simulink model "DinamicaNonLineare"  (R2020b)
settings: Solver=FixedStepDiscrete  StartTime=0.0  StopTime=inf  FixedStep=0.002  RelTol=1e-3
undefined symbols (not defined in the file or in its folder): DiscIntNeverNeededParam
libraries: simulink x4, sm_lib x4, nesl_utility x4, arduinolib x1
settings Model: SILPILModeSetting=veronly  ExtModeTrigDuration=2  Creator=Tommaso  LastModifiedBy=Tommaso
settings OptimizationCC: EnhancedBackFolding=on  PassReuseOutputArgsAs=Individual arguments  ZeroExternalMemoryAtStartup=off  ZeroInternalMemoryAtStartup=off  MaxStackSize=64  OptimizeBlockOrder=speed  DifferentSizesBufferReuse=on  OptimizationCustomize=off  EfficientTunableParamExpr=on
settings DebuggingCC: ParameterTunabilityLossMsg=error
settings HardwareCC: ProdBitPerInt=16  ProdBitPerPointer=16  ProdBitPerSizeT=16  ProdBitPerPtrDiffT=16  ProdLargestAtomicFloat=None  ProdWordSize=8  ProdHWDeviceType=Atmel->AVR
settings SFSimCC: MATLABDynamicMemAlloc=off
settings RTWCC: Description=Embedded Coder  SystemTargetFile=ert.tlc  HardwareBoard=Arduino Uno  TemplateMakefile=ert_default_tmf  Toolchain=Arduino AVR
settings CodeAppCC: ForceParamTrailComments=on  IgnoreCustomStorageClasses=off  OperatorAnnotations=on  SimulinkDataObjDesc=on  SFDataObjDesc=on  InsertBlockDesc=on
settings ERTTargetCC: SupportContinuousTime=on  SupportVariableSizeSignals=on  ExtModeStaticAllocSize=250
settings ExplorerConfigSet: InternalSimMechanicsExplorerSettings="<ExplorerConfiguration><canonicalview>default</canonicalview><AnimationSetting><BasePlaybackSpeed>1.0</BasePlaybackSpeed><PlaybackSpeedFactor>1.0</PlaybackSpeedFactor></AnimationSetting><TilePanel><TileInfo><Tiles Columns=\"1\" Count=\"1\" Rows=\"1\"><Column Weight=\"1\"/><Row Weight=\"1\"/><Tile Height=\"1\" Width=\"1\" X=\"0\" Y=\"0\"/></Tiles></TileInfo><SceneInfo><SceneViewer><BGColor><R>0.60000002384185791</R><G>0.60000002384185791</G><B>0.60000002384185791</B></BGColor><Camera><DoPerspective>off</DoPerspective><Position><X>-0.0398988425731658936</X><Y>-1.00037544965744019</Y><Z>0.00866047292947813574</Z></Position><Center><X>-0.0398988425731658936</X><Y>-0.000375449657440185547</Y><Z>0.00866047292947813574</Z></Center><Up><X>0</X><Y>-0</Y><Z>1</Z></Up><ViewLimDist>1</ViewLimDist><YLim>0.125903869368592103</YLim><XLim>0.183246225714683547</XLim></Camera></SceneViewer></SceneInfo></TilePanel><MechEditorPanel><Cameras/><GfxPanelCameraMap/><VideoCreator><PlaybackSpeedRatio>1.0</PlaybackSpeedRatio><FrameRate>30</FrameRate><VideoFormat>Motion JPEG AVI</VideoFormat><FrameSize>auto</FrameSize></VideoCreator></MechEditorPanel></ExplorerConfiguration>"

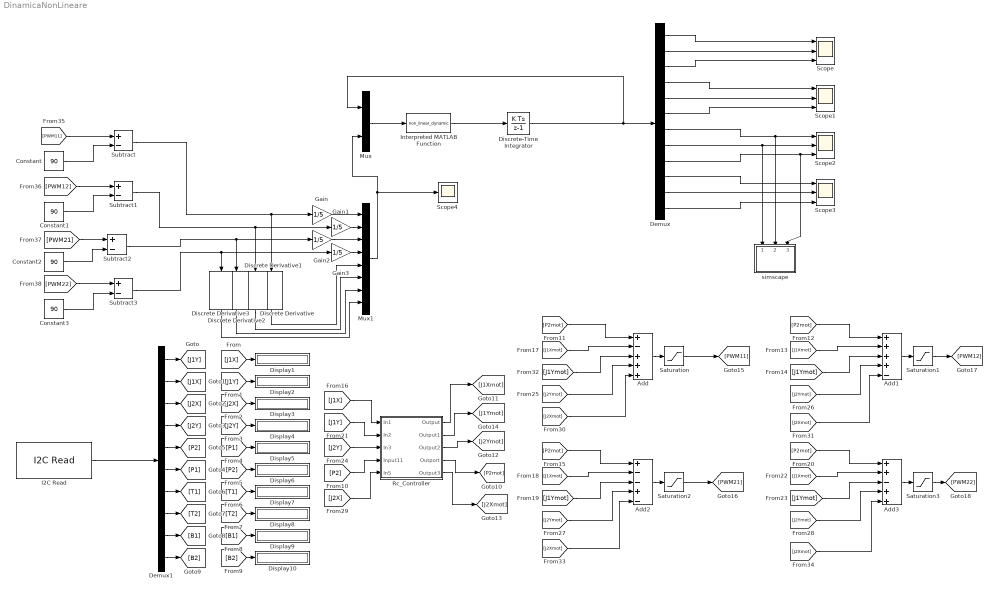
== system DinamicaNonLineare ==
  Add : Sum  Inputs=+-+++
  Add1 : Sum  Inputs=++++-
  Add2 : Sum  Inputs=+--+-
  Add3 : Sum  Inputs=++-++
  Constant{,1..3} (4 alike) : Constant  Value=90
  Demux : Demux  Outputs=12
  Demux1 : Demux  Outputs=10
  Discrete Derivative{,1..3} (4 alike) : simulink/Discrete/Discrete Derivative  gainval=1.0  ICPrevScaledInput=0.0  OutMin=[]  OutMax=[]  OutDataType=fixdt(1, 16)  OutScaling=2^-10  DoSatur=off
  Discrete-Time Integrator : DiscreteIntegrator  InitialCondition=[0,0,10,0,0,0,0,0,0,0,0,0]  SampleTime=-1  LimitOutput=on  UpperSaturationLimit=10^2  LowerSaturationLimit=-10^2  ICPrevOutput=DiscIntNeverNeededParam  ICPrevScaledInput=DiscIntNeverNeededParam
  Display{1..10} (10 alike) : Display
  Gain{,1..3} (4 alike) : Gain  Gain=1/5
  I2C Read : arduinolib/I2C Read  I2CModule=0  Mode=Master  SlaveAddress=08  SlaveByteOrder=BigEndian  Direction=Receiver  RegisterAddressMode=on  RegisterAddress=0  SlaveDataType=uint8  DataLength=10  NoAck=off  RepeatedStart=off  OutputStatus=off  blockPlatform=ARDUINO  SampleTime=1/500
      settings: SourceProductBaseCode=ARDUINO
  Interpreted MATLAB Function : MATLABFcn  MATLABFcn=non_linear_dynamic
  Mux : Mux  Inputs=2
  Mux1 : Mux  Inputs=8
  Rc_Controller : Subsystem
  Saturation{,1..3} (4 alike) : Saturate  UpperLimit=140  LowerLimit=90  LinearizeAsGain=off
  Scope{,1..3} (4 alike) : Scope  NumInputPorts=3
  Scope4 : Scope
  Subtract{,1..3} (4 alike) : Sum  Inputs=+-
  simscape : Subsystem
  wires:
  Mux/1 -> Interpreted MATLAB Function/1
  Discrete-Time Integrator/1 -> Demux/1, Mux/1
  Demux/1 -> Scope/1
  Demux/2 -> Scope/2
  Demux/3 -> Scope/3
  Demux/5 -> Scope1/2
  Demux/4 -> Scope1/1
  Demux/6 -> Scope1/3
  Demux/8 -> Scope2/2, simscape/1(Rot2)
  Demux/7 -> Scope2/1, simscape/2(Rot1)
  Mux1/1 -> Mux/2, Scope4/1
  Demux/11 -> Scope3/2
  Demux/10 -> Scope3/1
  Demux/12 -> Scope3/3
  [J1X] -> Rc_Controller/1(In1)
  [J1Xmot] -> Add/2
  [J1Ymot] -> Add2/3
  [B1] -> Display9/1
  [P2] -> Display6/1
  [P2mot] -> Add1/1
  [J2X] -> Display3/1
  [T2] -> Display8/1
  Demux1/9 -> [B1]
  Demux1/3 -> [J2X]
  Demux1/7 -> [T1]
  [T1] -> Display7/1
  [B2] -> Display10/1
  [J2Y] -> Display4/1
  Add3/1 -> Saturation3/1
  [J1Y] -> Display2/1
  Rc_Controller/3(Output2) -> [J2Ymot]
  Rc_Controller/4(Outport) -> [P2mot]
  Rc_Controller/1(Output) -> [J1Xmot]
  Saturation2/1 -> [PWM21]
  Demux1/2 -> [J1X]
  [P1] -> Display5/1
  [J1X] -> Display1/1
  [J2Xmot] -> Add1/5
  [J2Ymot] -> Add2/4
  [J2Xmot] -> Add/5
  [J2Ymot] -> Add/4
  Rc_Controller/5(Output3) -> [J2Xmot]
  I2C Read/1 -> Demux1/1
  [P2mot] -> Add3/1
  [J2Ymot] -> Add3/4
  [J1Xmot] -> Add2/2
  [J1Xmot] -> Add3/2
  [P2mot] -> Add/1
  Demux1/1 -> [J1Y]
  [P2mot] -> Add2/1
  [J1Xmot] -> Add1/2
  [J1Ymot] -> Add1/3
  Demux1/6 -> [P1]
  Demux1/4 -> [J2Y]
  Demux1/8 -> [T2]
  [J2Xmot] -> Add2/5
  Saturation1/1 -> [PWM12]
  Add/1 -> Saturation/1
  Demux1/10 -> [B2]
  [J2X] -> Rc_Controller/5(In5)
  [J2Xmot] -> Add3/5
  [J1Y] -> Rc_Controller/2(In2)
  [J1Ymot] -> Add/3
  Demux1/5 -> [P2]
  [J2Y] -> Rc_Controller/3(In3)
  [J2Ymot] -> Add1/4
  Add1/1 -> Saturation1/1
  [P2] -> Rc_Controller/4(Input11)
  [J1Ymot] -> Add3/3
  Rc_Controller/2(Output1) -> [J1Ymot]
  Add2/1 -> Saturation2/1
  Saturation/1 -> [PWM11]
  Saturation3/1 -> [PWM22]
  Gain/1 -> Mux1/1
  Gain2/1 -> Mux1/3
  Gain1/1 -> Mux1/2
  Gain3/1 -> Mux1/4
  Constant/1 -> Subtract/2
  [PWM11] -> Subtract/1
  Subtract/1 -> Gain/1, Discrete Derivative/1
  Constant1/1 -> Subtract1/2
  [PWM12] -> Subtract1/1
  Subtract1/1 -> Gain1/1, Discrete Derivative1/1
  Constant2/1 -> Subtract2/2
  [PWM21] -> Subtract2/1
  Subtract2/1 -> Discrete Derivative2/1, Gain2/1
  Constant3/1 -> Subtract3/2
  [PWM22] -> Subtract3/1
  Subtract3/1 -> Gain3/1, Discrete Derivative3/1
  Interpreted MATLAB Function/1 -> Discrete-Time Integrator/1
  Demux/9 -> simscape/3(Rot3), Scope2/3
  Discrete Derivative/1 -> Mux1/5
  Discrete Derivative1/1 -> Mux1/6
  Discrete Derivative2/1 -> Mux1/7
  Discrete Derivative3/1 -> Mux1/8

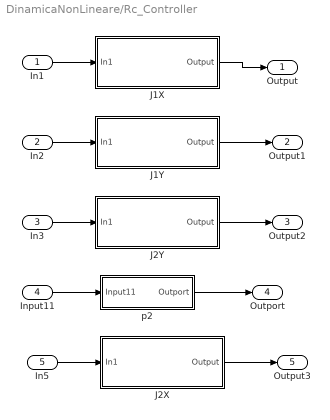
== system DinamicaNonLineare/Rc_Controller ==
  In1 : Inport
  In2 : Inport  Port=2
  In3 : Inport  Port=3
  Input11 : Inport  Port=4
  In5 : Inport  Port=5
  J1X : Subsystem
  J1Y : Subsystem
  J2X : Subsystem
  J2Y : Subsystem
  p2 : Subsystem
  Output : Outport
  Output1 : Outport  Port=2
  Output2 : Outport  Port=3
  Outport : Outport  Port=4
  Output3 : Outport  Port=5
  wires:
  Input11/1 -> p2/1(Input11)
  J2X/1(Output) -> Output3/1
  J1Y/1(Output) -> Output1/1
  In5/1 -> J2X/1(In1)
  J1X/1(Output) -> Output/1
  J2Y/1(Output) -> Output2/1
  In3/1 -> J2Y/1(In1)
  In1/1 -> J1X/1(In1)
  p2/1(Outport) -> Outport/1
  In2/1 -> J1Y/1(In1)

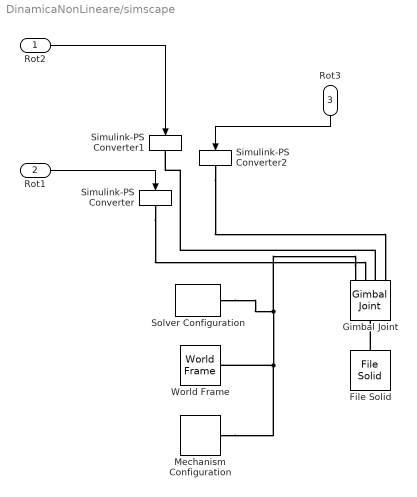
== system DinamicaNonLineare/simscape ==
  Rot2 : Inport
  Rot1 : Inport  Port=2
  Rot3 : Inport  Port=3
  File Solid : sm_lib/Body Elements/File Solid  ExtGeomFileName=C:\Users\Tommaso\università\Controlli Automatici\Nuovo\Relazione\GitRepo\MatlabSimulink\Ass_Global.STL  UnitType=Custom  ExtGeomFileUnits=mm  StepReaderType=HEX  ExportConvexHullGeometry=off  InertiaType=Custom  Mass=1  MassUnits=kg  CenterOfMass=[220 170 45]  CenterOfMassUnits=mm  MomentsOfInertia=[1 1 1]  MomentsOfInertiaUnits=kg*m^2  ProductsOfInertia=[0 0 0]  ProductsOfInertiaUnits=kg*m^2  BasedOnType=DensityFromFile  Density=1000  DensityUnits=kg/m^3  DoExposeReferenceFrame=off  SerializedFrames=<Frames><Frame><Id>Frame1</Id><Value><Name>F1</Name><Origin><Source>CenterOfMassFrame</Source><FeatureName></FeatureName></Origin><PrimaryAxis><DefinedDirection>+Z</DefinedDirection><Source>CenterOfMassFrame</Source><SourceDirection>+Z</SourceDirection><FeatureName></FeatureName></PrimaryAxis><SecondaryAxis><DefinedDirection>+X</DefinedDirection><Source>CenterOfMassFrame</Source><SourceDirection>+X</SourceDirection><FeatureName></FeatureName></SecondaryAxis></Value></Frame></Frames>  GraphicType=FromGeometry  MarkerShape=Sphere  MarkerSize=10  GraphicVisPropType=SimpleVisualProperties  GraphicDiffuseColor=[0.6 0.6 0.6]  GraphicSpecularColor=[0.5 0.5 0.5 1.0]  GraphicAmbientColor=[0.15 0.15 0.15 1.0]  GraphicEmissiveColor=[0.0 0.0 0.0 1.0]  GraphicShininess=75  GraphicOpacity=1.0
  Gimbal Joint : sm_lib/Joints/Gimbal Joint  JointMode=Normal  SenseConstraintForce=off  SenseConstraintForceX=off  SenseConstraintForceY=off  SenseConstraintForceZ=off  SenseConstraintTorque=off  SenseConstraintTorqueX=off  SenseConstraintTorqueY=off  SenseConstraintTorqueZ=off  SenseTotalForce=off  SenseTotalForceX=off  SenseTotalForceY=off  SenseTotalForceZ=off  SenseTotalTorque=off  SenseTotalTorqueX=off  SenseTotalTorqueY=off  SenseTotalTorqueZ=off  CompositeWrenchDir=FollowerOnBase  CompositeWrenchFrame=BaseFrame  RxEquilibriumPosition=0  RxEquilibriumPositionUnits=deg  RxSpringStiffness=0  RxSpringStiffnessUnits=N*m/deg  RxDampingCoefficient=0  RxDampingCoefficientUnits=N*m/(deg/s)  RxTorqueActuationMode=ComputedTorque  RxMotionActuationMode=InputMotion  RxSensePosition=off  RxSenseVelocity=off  RxSenseAcceleration=off  RxSenseTorqueForce=off  RxSenseLowerLimitTorqueForce=off  RxSenseUpperLimitTorqueForce=off  RxLowerLimitSpecify=off  RxLowerLimitBound=-90  RxLowerLimitBoundUnits=deg  RxLowerLimitStiffness=1e4  RxLowerLimitStiffnessUnits=N*m/deg  RxLowerLimitDamping=10  RxLowerLimitDampingUnits=N*m/(deg/s)  RxLowerLimitTransitionRegionWidth=0.1  RxLowerLimitTransitionRegionWidthUnits=deg  RxUpperLimitSpecify=off  RxUpperLimitBound=90  RxUpperLimitBoundUnits=deg  RxUpperLimitStiffness=1e4  RxUpperLimitStiffnessUnits=N*m/deg  RxUpperLimitDamping=10  RxUpperLimitDampingUnits=N*m/(deg/s)  RxUpperLimitTransitionRegionWidth=0.1  RxUpperLimitTransitionRegionWidthUnits=deg  RxPositionTargetSpecify=off  RxPositionTargetPriority=High  RxPositionTargetValue=0  RxPositionTargetValueUnits=deg  RxVelocityTargetSpecify=off  RxVelocityTargetPriority=High  RxVelocityTargetValue=0  RxVelocityTargetValueUnits=deg/s  RyEquilibriumPosition=0  RyEquilibriumPositionUnits=deg  RySpringStiffness=0  RySpringStiffnessUnits=N*m/deg  RyDampingCoefficient=0  RyDampingCoefficientUnits=N*m/(deg/s)  RyTorqueActuationMode=ComputedTorque  RyMotionActuationMode=InputMotion  RySensePosition=off  RySenseVelocity=off  RySenseAcceleration=off  RySenseTorqueForce=off  RySenseLowerLimitTorqueForce=off  RySenseUpperLimitTorqueForce=off  RyLowerLimitSpecify=off  RyLowerLimitBound=-90  RyLowerLimitBoundUnits=deg  RyLowerLimitStiffness=1e4  RyLowerLimitStiffnessUnits=N*m/deg  RyLowerLimitDamping=10  RyLowerLimitDampingUnits=N*m/(deg/s)  RyLowerLimitTransitionRegionWidth=0.1  RyLowerLimitTransitionRegionWidthUnits=deg  RyUpperLimitSpecify=off  RyUpperLimitBound=90  RyUpperLimitBoundUnits=deg  RyUpperLimitStiffness=1e4  RyUpperLimitStiffnessUnits=N*m/deg  RyUpperLimitDamping=10  RyUpperLimitDampingUnits=N*m/(deg/s)  RyUpperLimitTransitionRegionWidth=0.1  RyUpperLimitTransitionRegionWidthUnits=deg  RyPositionTargetSpecify=off  RyPositionTargetPriority=High  RyPositionTargetValue=0  RyPositionTargetValueUnits=deg  RyVelocityTargetSpecify=off  RyVelocityTargetPriority=High  RyVelocityTargetValue=0  RyVelocityTargetValueUnits=deg/s  RzEquilibriumPosition=0  RzEquilibriumPositionUnits=deg  RzSpringStiffness=0  RzSpringStiffnessUnits=N*m/deg  RzDampingCoefficient=0  RzDampingCoefficientUnits=N*m/(deg/s)  RzTorqueActuationMode=ComputedTorque  RzMotionActuationMode=InputMotion  RzSensePosition=off  RzSenseVelocity=off  RzSenseAcceleration=off  RzSenseTorqueForce=off  RzSenseLowerLimitTorqueForce=off  RzSenseUpperLimitTorqueForce=off  RzLowerLimitSpecify=off  RzLowerLimitBound=-90  RzLowerLimitBoundUnits=deg  RzLowerLimitStiffness=1e4  RzLowerLimitStiffnessUnits=N*m/deg  RzLowerLimitDamping=10  RzLowerLimitDampingUnits=N*m/(deg/s)  RzLowerLimitTransitionRegionWidth=0.1  RzLowerLimitTransitionRegionWidthUnits=deg  RzUpperLimitSpecify=off  RzUpperLimitBound=90  RzUpperLimitBoundUnits=deg  RzUpperLimitStiffness=1e4  RzUpperLimitStiffnessUnits=N*m/deg  RzUpperLimitDamping=10  RzUpperLimitDampingUnits=N*m/(deg/s)  RzUpperLimitTransitionRegionWidth=0.1  RzUpperLimitTransitionRegionWidthUnits=deg  RzPositionTargetSpecify=off  RzPositionTargetPriority=High  RzPositionTargetValue=0  RzPositionTargetValueUnits=deg  RzVelocityTargetSpecify=off  RzVelocityTargetPriority=High  RzVelocityTargetValue=0  RzVelocityTargetValueUnits=deg/s
  Mechanism Configuration : sm_lib/Utilities/Mechanism Configuration  UniformGravity=Constant  GravityVector=[0 0 -9.80665]  GravityVectorUnits=m/s^2  GravityUnits=m/s^2  LinearizationDelta=0.001  JointModeTransitionNonlinearIterations=2
  Simulink-PS Converter : nesl_utility/Simulink-PS Converter  PhysicalDomain=network_engine_domain  SubClassName=ps_input  LeftPortType=input  RightPortType=output  PseudoPeriodic=off  Frequencies=[]  NoiseDistribution=none  NoiseParameters=[]  Unit=rad  AffineConversion=off  FilteringAndDerivatives=zero  SimscapeFilterOrder=1  InputFilterTimeConstant=0.001  UdotUserProvided=0
  Simulink-PS Converter1 : nesl_utility/Simulink-PS Converter  PhysicalDomain=network_engine_domain  SubClassName=ps_input  LeftPortType=input  RightPortType=output  PseudoPeriodic=off  Frequencies=[]  NoiseDistribution=none  NoiseParameters=[]  Unit=rad  AffineConversion=off  FilteringAndDerivatives=zero  SimscapeFilterOrder=1  InputFilterTimeConstant=0.001  UdotUserProvided=0
  Simulink-PS Converter2 : nesl_utility/Simulink-PS Converter  PhysicalDomain=network_engine_domain  SubClassName=ps_input  LeftPortType=input  RightPortType=output  PseudoPeriodic=off  Frequencies=[]  NoiseDistribution=none  NoiseParameters=[]  Unit=rad  AffineConversion=off  FilteringAndDerivatives=zero  SimscapeFilterOrder=1  InputFilterTimeConstant=0.001  UdotUserProvided=0
  Solver Configuration : nesl_utility/Solver Configuration  PhysicalDomain=network_engine_domain  SubClassName=solver  LeftPortType=input  RightPortType=generic  Tones=[]  Harmonics=[]  SimulateNoise=off  Profile=off  UseLocalSampling=off  EnableSwitchedLinearOptims=on  FrequencyDomain=off  UseCCode=off  RelTol=0.001  AbsTol=1e-06  MinStep=1e-09  ToWorkspace=off  RevertToSquareIcSolve=off  NumHomotopyIterations=100  PhasorMode=off  PhasorModeNumHarmonics=1  DoDC=off  ResidualTolerance=1e-09  UseLocalSolver=off  LocalSolverChoice=NE_BACKWARD_EULER_ADVANCER  LocalSolverSampleTime=0.001  DoFixedCost=off  MaxNonlinIter=3  MaxModeIter=2  ComputeImpulses=off  ImpulseIterations=2  LinearAlgebra=auto  EquationFormulation=NE_TIME_EF  DelaysMemoryBudget=1024  AutomaticFiltering=on  FilteringTimeConstant=0.001  PartitionStorageMethod=AS_NEEDED  PartitionMemoryBudget=1024  PartitionMethod=ROBUST
  World Frame : sm_lib/Frames and Transforms/World Frame
  wires:
  Rot2/1 -> Simulink-PS Converter1/1
  Rot3/1 -> Simulink-PS Converter2/1
  Rot1/1 -> Simulink-PS Converter/1
  connections:
  Gimbal Joint/LConn3 -- Simulink-PS Converter1/RConn1
  Gimbal Joint/LConn1 -- World Frame/RConn1 -- Mechanism Configuration/RConn1 -- Solver Configuration/RConn1
  File Solid/LConn1 -- Gimbal Joint/RConn1
  Simulink-PS Converter/RConn1 -- Gimbal Joint/LConn2
  Simulink-PS Converter2/RConn1 -- Gimbal Joint/LConn4

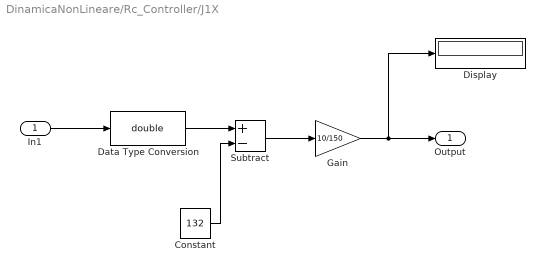
== system DinamicaNonLineare/Rc_Controller/J1X ==
  In1 : Inport
  Constant : Constant  Value=132
  Data Type Conversion : DataTypeConversion  OutDataTypeStr=double
  Display : Display
  Gain : Gain  Gain=10/150
  Subtract : Sum  Inputs=+-
  Output : Outport
  wires:
  Gain/1 -> Display/1, Output/1
  Constant/1 -> Subtract/2
  In1/1 -> Data Type Conversion/1
  Data Type Conversion/1 -> Subtract/1
  Subtract/1 -> Gain/1

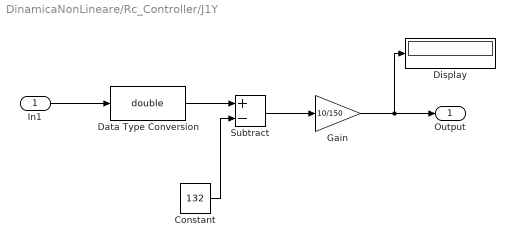
== system DinamicaNonLineare/Rc_Controller/J1Y ==
  In1 : Inport
  Constant : Constant  Value=132
  Data Type Conversion : DataTypeConversion  OutDataTypeStr=double
  Display : Display
  Gain : Gain  Gain=10/150
  Subtract : Sum  Inputs=+-
  Output : Outport
  wires:
  Gain/1 -> Display/1, Output/1
  Constant/1 -> Subtract/2
  In1/1 -> Data Type Conversion/1
  Data Type Conversion/1 -> Subtract/1
  Subtract/1 -> Gain/1

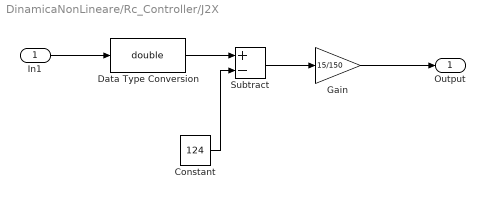
== system DinamicaNonLineare/Rc_Controller/J2X ==
  In1 : Inport
  Constant : Constant  Value=124
  Data Type Conversion : DataTypeConversion  OutDataTypeStr=double
  Gain : Gain  Gain=15/150
  Subtract : Sum  Inputs=+-
  Output : Outport
  wires:
  Gain/1 -> Output/1
  Constant/1 -> Subtract/2
  In1/1 -> Data Type Conversion/1
  Data Type Conversion/1 -> Subtract/1
  Subtract/1 -> Gain/1

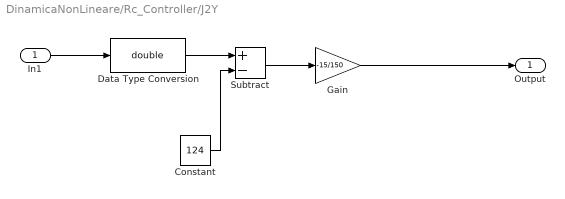
== system DinamicaNonLineare/Rc_Controller/J2Y ==
  In1 : Inport
  Constant : Constant  Value=124
  Data Type Conversion : DataTypeConversion  OutDataTypeStr=double
  Gain : Gain  Gain=-15/150
  Subtract : Sum  Inputs=+-
  Output : Outport
  wires:
  Gain/1 -> Output/1
  Constant/1 -> Subtract/2
  In1/1 -> Data Type Conversion/1
  Data Type Conversion/1 -> Subtract/1
  Subtract/1 -> Gain/1

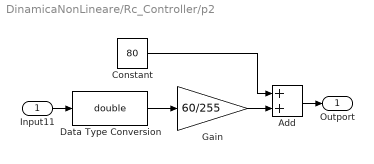
== system DinamicaNonLineare/Rc_Controller/p2 ==
  Input11 : Inport
  Add : Sum
  Constant : Constant  Value=80  OutDataTypeStr=double
  Data Type Conversion : DataTypeConversion  OutDataTypeStr=double
  Gain : Gain  Gain=60/255
  Outport : Outport
  wires:
  Gain/1 -> Add/2
  Data Type Conversion/1 -> Gain/1
  Add/1 -> Outport/1
  Constant/1 -> Add/1
  Input11/1 -> Data Type Conversion/1
